simulink model "acionamento"  (R2015a)
settings: Solver=ode45  StartTime=0.0  StopTime=6.0  RelTol=1e-3
values from neighbouring files (symbols this model uses):
  Ts = 2e-05    [script_acionamento.m]
libraries: powerlib x4, powerlib_meascontrol x3
settings Model: Creator=range  LastModifiedBy=range

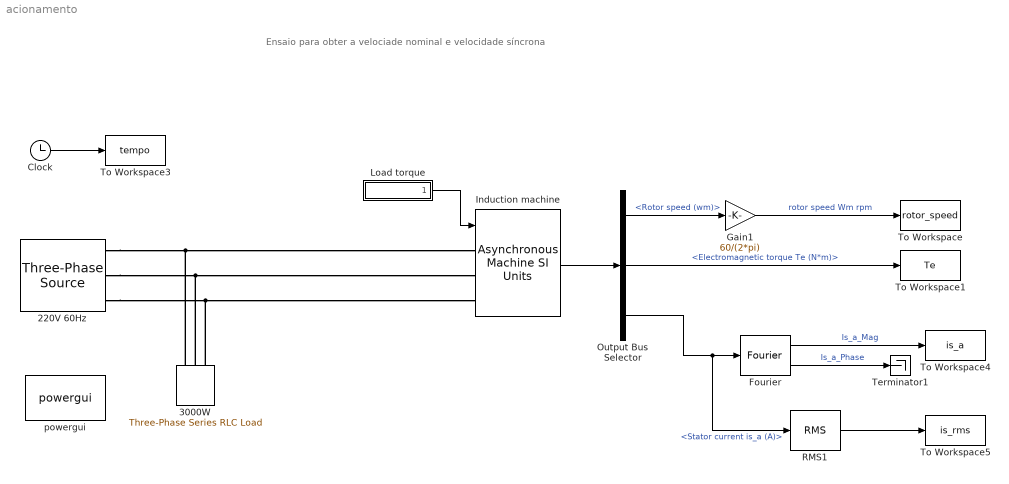
== system acionamento ==
  note: Ensaio para obter a velociade nominal e velocidade síncrona
  220V 60Hz : powerlib/Electrical Sources/Three-Phase Source  Voltage=220  PhaseAngle=0  Frequency=60  InternalConnection=Yg  SpecifyImpedance=off  Resistance=0.5  Inductance=0.1e-3  ShortCircuitLevel=0  BaseVoltage=0  XRratio=0  BusType=swing  Pref=0  Qref=0  Qmin=-inf  Qmax=inf
  3000W : powerlib/Elements/Three-Phase Series RLC Load  LConnTagsString=A|B|C  Configuration=Y (grounded)  NominalVoltage=220  NominalFrequency=60  ActivePower=30000  InductivePower=0  CapacitivePower=0  Measurements=None  LoadType=constant Z
  Clock : Clock
  Fourier : powerlib_meascontrol/Measurements/Fourier  Freq=60  n=1  InInit=[0, 0]  Ts=Ts
  Gain1 : Gain  Gain=60/(2*pi)
  Induction machine : powerlib/Machines/Asynchronous Machine SI Units  RotorType=Squirrel-cage  PresetModel=No  MechanicalLoad=Torque Tm  ShowDetailedParameters=on  ReferenceFrame=Stationary  Units=SI  MeasurementBus=off  NominalParameters=[2238,220,60]  Stator=[0.435,0.002]  Rotor=[0.816,0.002]  Cage1=[ 0.022 0.226/377]  Cage2=[ 0.022 0.226/377]  Lm=69.31e-3  Mechanical=[0.089,0.005,2]  PolePairs=2  InitialConditions=[1,0,0,0,0,0,0,0]  SimulateSaturation=off  Saturation=[0 0;0 0]  LoadFlowParameters=0  TsPowergui=0  TsBlock=-1  IterativeModel=Trapezoidal non iterative  Pmec=0
  Load torque : Subsystem
  Output Bus Selector : BusSelector  OutputSignals=Mechanical.Rotor speed (wm),Mechanical.Electromagnetic torque Te (N*m),Stator measurements.Stator current is_a (A)
  RMS1 : powerlib_meascontrol/Measurements/RMS  TrueRMS=on  Freq=60  RMSInit=0  Ts=Ts
  Terminator1 : Terminator
  To Workspace : ToWorkspace  VariableName=rotor_speed  SampleTime=Ts
  To Workspace1 : ToWorkspace  VariableName=Te  SampleTime=Ts
  To Workspace3 : ToWorkspace  VariableName=tempo  SampleTime=Ts
  To Workspace4 : ToWorkspace  VariableName=is_a  SampleTime=Ts
  To Workspace5 : ToWorkspace  VariableName=is_rms  SampleTime=Ts
  powergui : powerlib/powergui  Priority=2  SimulationMode=Discrete  SolverType=Tustin/Backward Euler (TBE)  SampleTime=Ts  frequency=60  SPID=off  DisableSnubberDevices=on  DisableRonSwitches=off  DisableVfSwitches=off  SwTol=0  DisplayEquations=off  Interpol=off  methode=off  Ts=0  FunctionMessages=off  echomessages=off  HookPort=off  EnableUseOfTLC=off  x0status=blocks  frequencyindice=60  Pbase=100e6  ErrMax=1e-4  Iterations=50  UnitsV=kV  UnitsW=MW  buscounter=0  RestoreLinks=warning  ResistiveCurrentMeasurement=off  Frange=[0:2:500]  Ylog=off  Xlog=on  ShowGrid=off  save=off  variable=ZData  structure=0  ZoomFFT=on  StartTime=0.0  cycles=1  DisplayStyle=1  fundamental=60  FreqAxis=off  MaxFrequency=1000  frequencyindicesteady=1  RmsSteady=1  display=off
  wires:
  Induction machine/1 -> Output Bus Selector/1
  Load torque/1(" ") -> Induction machine/1
  Output Bus Selector/1 -> Gain1/1  "<Rotor speed (wm)>"
  Gain1/1 -> To Workspace/1  "rotor speed Wm rpm"
  Output Bus Selector/2 -> To Workspace1/1  "<Electromagnetic torque Te (N*m)>"
  Clock/1 -> To Workspace3/1
  Output Bus Selector/3 -> RMS1/1, Fourier/1  "<Stator current is_a (A)>"
  Fourier/2 -> Terminator1/1  "Is_a_Phase"
  Fourier/1 -> To Workspace4/1  "Is_a_Mag"
  RMS1/1 -> To Workspace5/1
  connections:
  220V 60Hz/RConn1 -- 3000W/LConn1 -- Induction machine/LConn1
  220V 60Hz/RConn2 -- Induction machine/LConn2 -- 3000W/LConn2
  220V 60Hz/RConn3 -- Induction machine/LConn3 -- 3000W/LConn3

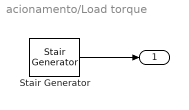
== system acionamento/Load torque ==
  Stair Generator : powerlib_meascontrol/Pulse & Signal Generators/Stair Generator  t=[0. 2.]  e=[0. 6.8]  Ts=Ts
  " " : Outport
  wires:
  Stair Generator/1 -> " "/1
